simulink model "PMSMEstimate"  (R2016a)
settings: Solver=ode4  StartTime=0.0  StopTime=3  FixedStep=1e-04  RelTol=1e-3
libraries: powerlib x7, dsparch4 x7, powerlib_meascontrol x3, simulink x1
settings Model: Creator=B210b  LastModifiedBy=B210b

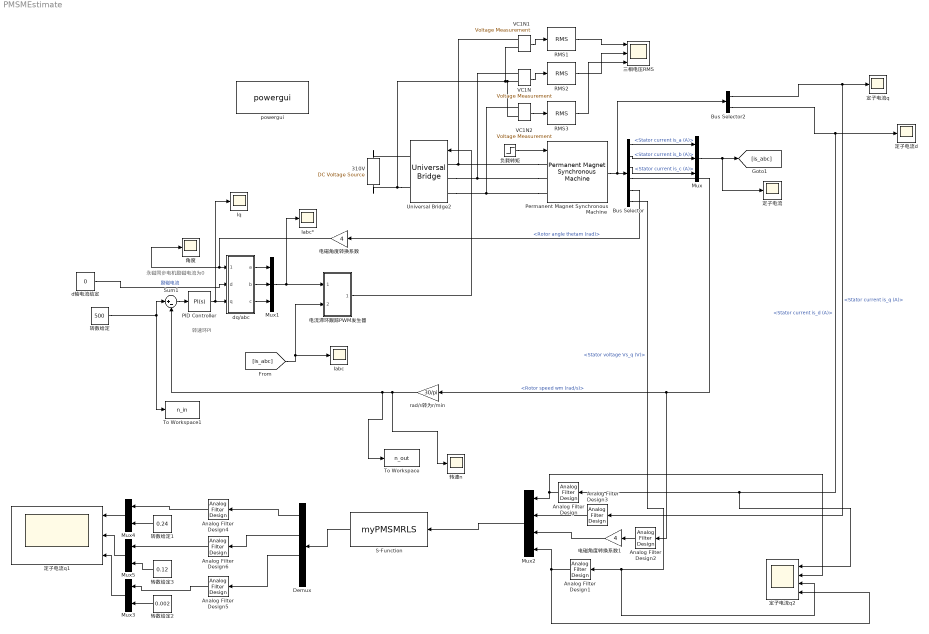
== system PMSMEstimate ==
  note: 转速环PI
  note: 永磁同步电机励磁电流为0
  310V : powerlib/Electrical Sources/DC Voltage Source  Amplitude=310  Measurements=None
  Analog Filter Design{,1..3} (4 alike) : dsparch4/Analog Filter Design  method=Butterworth  filttype=Lowpass  N=8  Wlo=50  Whi=80  Rp=2  Rs=40
  Analog Filter Design4 : dsparch4/Analog Filter Design  method=Butterworth  filttype=Lowpass  N=8  Wlo=20  Whi=80  Rp=2  Rs=40
  Analog Filter Design5 : dsparch4/Analog Filter Design  method=Butterworth  filttype=Lowpass  N=8  Wlo=20  Whi=80  Rp=2  Rs=40
  Analog Filter Design6 : dsparch4/Analog Filter Design  method=Butterworth  filttype=Lowpass  N=8  Wlo=20  Whi=80  Rp=2  Rs=40
  Bus Selector : BusSelector  OutputSignals=Stator current is_a (A),Stator current is_b (A),Stator current is_c (A),Rotor speed wm (rad/s),Rotor angle thetam (rad),Stator voltage Vs_q (V)
  Bus Selector2 : BusSelector  OutputSignals=Stator current is_q (A),Stator current is_d (A)
  Demux : Demux
  Iabc : Scope
  Iabc* : Scope
  Iq : Scope
  Mux : Mux  Inputs=3
  Mux1 : Mux  Inputs=3
  Mux2 : Mux
  Mux3 : Mux  Inputs=2
  Mux4 : Mux  Inputs=2
  Mux5 : Mux  Inputs=2
  PID Controller : simulink/Continuous/PID Controller  Controller=PI  TimeDomain=Continuous-time  SampleTime=-1  IntegratorMethod=Forward Euler  FilterMethod=Forward Euler  Form=Parallel  UseFilter=on  ControllerParametersSource=internal  P=0.05  I=8  D=0  N=100  InitialConditionSource=internal  InitialConditionForIntegrator=0  InitialConditionForFilter=0  ExternalReset=none  LimitOutput=off  UpperSaturationLimit=200  LowerSaturationLimit=-inf  LinearizeAsGain=on  AntiWindupMode=none  Kb=1  TrackingMode=off  Kt=1  PParamMin=[]  PParamMax=[]  IParamMin=[]  IParamMax=[]  DParamMin=[]  DParamMax=[]  NParamMin=[]  NParamMax=[]  KbParamMin=[]  KbParamMax=[]  KtParamMin=[]  KtParamMax=[]  POutMin=[]  POutMax=[]  IOutMin=[]  IOutMax=[]  DOutMin=[]  DOutMax=[]  NOutMin=[]  NOutMax=[]  KbOutMin=[]  KbOutMax=[]  KtOutMin=[]  KtOutMax=[]  IntegratorOutMin=[]  IntegratorOutMax=[]  FilterOutMin=[]  FilterOutMax=[]  SumOutMin=[]  SumOutMax=[]  SumI1OutMin=[]  SumI1OutMax=[]  SumI2OutMin=[]  SumI2OutMax=[]  SumI3OutMin=[]  SumI3OutMax=[]  SumDOutMin=[]  SumDOutMax=[]  SaturationOutMin=[]  SaturationOutMax=[]  IntegratorContinuousStateAttributes=''  IntegratorStateMustResolveToSignalObject=off  IntegratorRTWStateStorageClass=Auto  FilterContinuousStateAttributes=''  FilterStateMustResolveToSignalObject=off  FilterRTWStateStorageClass=Auto  DifferentiatorICPrevScaledInput=0  DifferentiatorOutMin=[]  DifferentiatorOutMax=[]
  Permanent Magnet Synchronous Machine : powerlib/Machines/Permanent Magnet Synchronous Machine  NbPhases=3  FluxDistribution=Sinusoidal  RotorType=Salient-pole  MechanicalLoad=Torque Tm  PresetModel=No  ShowDetailedParameters=on  MeasurementBus=off  Resistance=0.24  Inductance=8.5e-3  dqInductances=[0.002 0.002]  La=0.02682  MachineConstant=Flux linkage established by magnets (V.s)  Flux=0.12  VoltageCst=87.0624  TorqueCst=0.72  Flat=120  Mechanical=[0.00048 0.008 4 0]  PolePairs=2  InitialConditions=[0,0, 0,0]  InitialConditions5ph=[0 0 0 0 0 0]  TsPowergui=0  TsBlock=-1  RefAngle=Aligned with phase A axis (original Park)
  RMS1 : powerlib_meascontrol/Measurements/RMS  TrueRMS=on  Freq=100  RMSInit=0  Ts=0
  RMS2 : powerlib_meascontrol/Measurements/RMS  TrueRMS=on  Freq=100  RMSInit=0  Ts=0
  RMS3 : powerlib_meascontrol/Measurements/RMS  TrueRMS=on  Freq=100  RMSInit=0  Ts=0
  S-Function : S-Function  FunctionName=myPMSMRLS  SFunctionDeploymentMode=off  EnableBusSupport=off
  Sum1 : Sum  Inputs=|+-
  To Workspace : ToWorkspace  VariableName=n_out  SampleTime=-1
  To Workspace1 : ToWorkspace  VariableName=n_in  SampleTime=-1
  Universal Bridge2 : powerlib/Power Electronics/Universal Bridge  Arms=3  SnubberResistance=1e5  SnubberCapacitance=inf  Device=IGBT / Diodes  Ron=1e-3  Lon=0  ForwardVoltages="[  0  0  ]"  ForwardVoltage=0  GTOparameters=[ 10e-6 , 20e-6 ]  IGBTparameters=[ 1e-6 , 2e-6 ]  Measurements=None  Measurements_2=None  converterType=Rectifier
  VC1N : powerlib/Measurements/Voltage Measurement  PhasorSimulation=off  OutputType=Complex  PSBequivalent=0
  VC1N1 : powerlib/Measurements/Voltage Measurement  PhasorSimulation=off  OutputType=Complex  PSBequivalent=0
  VC1N2 : powerlib/Measurements/Voltage Measurement  PhasorSimulation=off  OutputType=Complex  PSBequivalent=0
  dq/abc : Subsystem
  d轴电流给定 : Constant  Value=0
  powergui : powerlib/powergui  SimulationMode=Continuous  SolverType=Tustin/Backward Euler (TBE)  SampleTime=0.00001  frequency=50  SPID=on  DisableSnubberDevices=off  DisableRonSwitches=off  DisableVfSwitches=off  SwTol=0  DisplayEquations=off  Interpol=off  ExternalGateDelay=off  methode=off  Ts=100  FunctionMessages=off  echomessages=off  HookPort=off  EnableUseOfTLC=off  x0status=zero  frequencyindice=0  Pbase=100e6  ErrMax=1e-4  Iterations=50  UnitsV=kV  UnitsW=MW  buscounter=0  RestoreLinks=warning  ResistiveCurrentMeasurement=off  Frange=[0:2:500]  Ylog=off  Xlog=on  ShowGrid=off  save=off  variable=ZData  structure=0  ZoomFFT=on  StartTime=0.0  cycles=1  DisplayStyle=1  fundamental=60  FreqAxis=off  MaxFrequency=1000  frequencyindicesteady=1  RmsSteady=1  display=off
  rad/s转为r/min : Gain  Gain=30/pi
  三相电压RMS : Scope  NumInputPorts=3
  定子电流 : Scope
  定子电流d : Scope
  定子电流q : Scope
  定子电流q1 : Scope  NumInputPorts=3
  定子电流q2 : Scope  NumInputPorts=4
  电流滞环跟踪PWM发生器 : Subsystem
  电磁角度转换系数 : Gain  Gain=4
  电磁角度转换系数1 : Gain  Gain=4
  角度 : Scope
  负载转矩 : Step  Time=0.02  Before=4  After=10  SampleTime=0
  转数给定 : Constant  Value=500
  转数给定1 : Constant  Value=0.24
  转数给定2 : Constant  Value=0.002
  转数给定3 : Constant  Value=0.12
  转速n : Scope
  wires:
  负载转矩/1 -> Permanent Magnet Synchronous Machine/1
  Permanent Magnet Synchronous Machine/1 -> Bus Selector2/1, Bus Selector/1
  Bus Selector/1 -> Mux/1  "<Stator current is_a (A)>"
  Bus Selector/2 -> Mux/2  "<Stator current is_b (A)>"
  Bus Selector/3 -> Mux/3  "<Stator current is_c (A)>"
  Bus Selector/4 -> Analog Filter Design2/1, rad/s转为r/min/1  "<Rotor speed wm (rad/s)>"
  Bus Selector/5 -> 电磁角度转换系数/1  "<Rotor angle thetam (rad)>"
  转数给定/1 -> Sum1/1, To Workspace1/1
  d轴电流给定/1 -> dq/abc/2(d)  "励磁电流"
  Mux/1 -> 定子电流/1, [is_abc]
  dq/abc/1(a) -> Mux1/1
  dq/abc/2(b) -> Mux1/2
  dq/abc/3(c) -> Mux1/3
  Mux1/1 -> Iabc*/1, 电流滞环跟踪PWM发生器/1(Iabc*)
  [is_abc] -> Iabc/1, 电流滞环跟踪PWM发生器/2(Iabc)
  电磁角度转换系数/1 -> 角度/1, dq/abc/1(theta)
  电流滞环跟踪PWM发生器/1(pulse) -> Universal Bridge2/1
  Sum1/1 -> PID Controller/1
  PID Controller/1 -> Iq/1, dq/abc/3(q)
  Bus Selector2/1 -> Analog Filter Design3/1, 定子电流q/1  "<Stator current is_q (A)>"
  Bus Selector2/2 -> 定子电流q2/1, Analog Filter Design/1, 定子电流d/1  "<Stator current is_d (A)>"
  rad/s转为r/min/1 -> To Workspace/1, Sum1/2, 转速n/1
  VC1N/1 -> RMS2/1
  VC1N1/1 -> RMS1/1
  RMS1/1 -> 三相电压RMS/1
  RMS2/1 -> 三相电压RMS/2
  VC1N2/1 -> RMS3/1
  RMS3/1 -> 三相电压RMS/3
  Mux2/1 -> S-Function/1
  电磁角度转换系数1/1 -> Mux2/3
  Bus Selector/6 -> 定子电流q2/3, Analog Filter Design1/1  "<Stator voltage Vs_q (V)>"
  Demux/1 -> Analog Filter Design4/1
  Demux/2 -> Analog Filter Design6/1
  Demux/3 -> Analog Filter Design5/1
  S-Function/1 -> Demux/1
  Analog Filter Design/1 -> Mux2/1, 定子电流q2/2
  Analog Filter Design3/1 -> Mux2/2
  Analog Filter Design2/1 -> 电磁角度转换系数1/1
  Analog Filter Design1/1 -> Mux2/4, 定子电流q2/4
  Mux4/1 -> 定子电流q1/1
  Mux5/1 -> 定子电流q1/2
  Mux3/1 -> 定子电流q1/3
  Analog Filter Design4/1 -> Mux4/1
  转数给定1/1 -> Mux4/2
  转数给定3/1 -> Mux5/2
  转数给定2/1 -> Mux3/2
  Analog Filter Design5/1 -> Mux3/1
  Analog Filter Design6/1 -> Mux5/1
  connections:
  Universal Bridge2/RConn2 -- 310V/LConn1 -- VC1N2/LConn2 -- VC1N/LConn2 -- VC1N1/LConn2
  Permanent Magnet Synchronous Machine/LConn1 -- Universal Bridge2/LConn1 -- VC1N1/LConn1
  Permanent Magnet Synchronous Machine/LConn3 -- Universal Bridge2/LConn3 -- VC1N2/LConn1
  Permanent Magnet Synchronous Machine/LConn2 -- Universal Bridge2/LConn2 -- VC1N/LConn1
  310V/RConn1 -- Universal Bridge2/RConn1

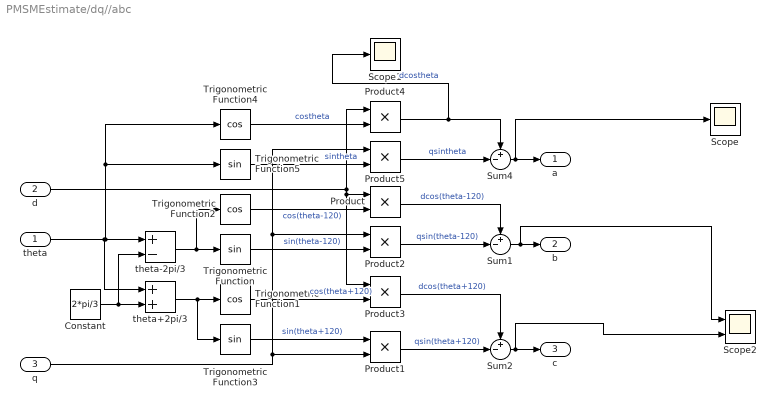
== system PMSMEstimate/dq//abc ==
  theta : Inport
  d : Inport  Port=2
  q : Inport  Port=3
  Constant : Constant  Value=2*pi/3
  Product{,1..5} (6 alike) : Product
  Scope : Scope
  Scope1 : Scope
  Scope2 : Scope  NumInputPorts=2
  Sum1 : Sum  Inputs=+-|
  Sum2 : Sum  Inputs=+-|
  Sum4 : Sum  Inputs=+-|
  Trigonometric Function : Trigonometry
  Trigonometric Function1 : Trigonometry  Operator=cos
  Trigonometric Function2 : Trigonometry  Operator=cos
  Trigonometric Function3 : Trigonometry
  Trigonometric Function4 : Trigonometry  Operator=cos
  Trigonometric Function5 : Trigonometry
  theta+2pi/3 : Sum
  theta-2pi/3 : Sum  Inputs=+-
  a : Outport
  b : Outport  Port=2
  c : Outport  Port=3
  wires:
  Trigonometric Function5/1 -> Product5/2  "sintheta"
  Product/1 -> Sum1/1  "dcos(theta-120)"
  Trigonometric Function1/1 -> Product3/2  "cos(theta+120)"
  Product3/1 -> Sum2/1  "dcos(theta+120)"
  d/1 -> Product/1, Product3/1, Product4/1
  Constant/1 -> theta+2pi/3/2, theta-2pi/3/2
  theta/1 -> Trigonometric Function4/1, Trigonometric Function5/1, theta-2pi/3/1, theta+2pi/3/1
  theta+2pi/3/1 -> Trigonometric Function3/1, Trigonometric Function1/1
  q/1 -> Product5/1, Product2/1, Product1/2
  Trigonometric Function/1 -> Product2/2  "sin(theta-120)"
  Product4/1 -> Scope1/1, Sum4/1  "dcostheta"
  Product5/1 -> Sum4/2  "qsintheta"
  theta-2pi/3/1 -> Trigonometric Function2/1, Trigonometric Function/1
  Product1/1 -> Sum2/2  "qsin(theta+120)"
  Trigonometric Function2/1 -> Product/2  "cos(theta-120)"
  Sum4/1 -> Scope/1, a/1
  Sum1/1 -> Scope2/1, b/1
  Trigonometric Function4/1 -> Product4/2  "costheta"
  Trigonometric Function3/1 -> Product1/1  "sin(theta+120)"
  Product2/1 -> Sum1/2  "qsin(theta-120)"
  Sum2/1 -> Scope2/2, c/1

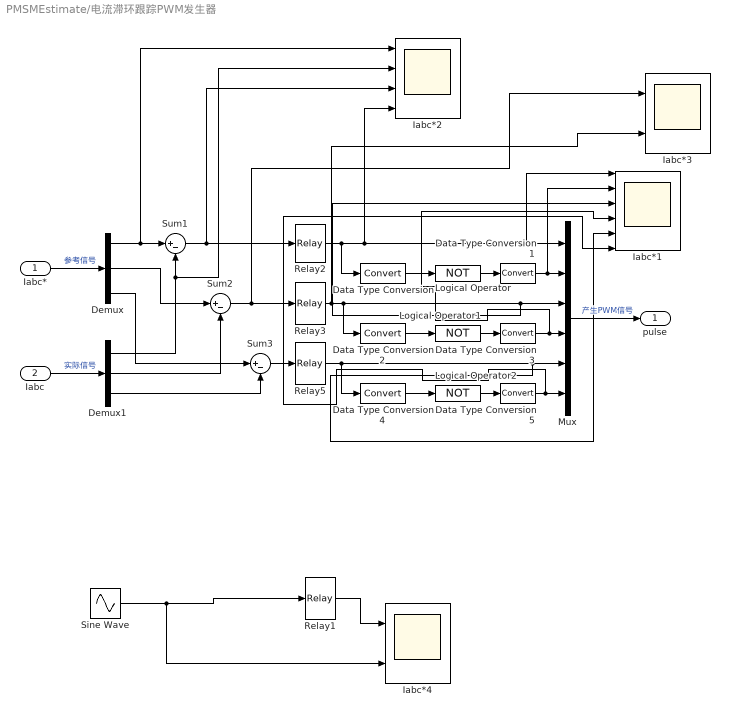
== system PMSMEstimate/电流滞环跟踪PWM发生器 ==
  Iabc* : Inport
  Iabc : Inport  Port=2
  Data Type Conversion{,1..5} (6 alike) : DataTypeConversion
  Demux : Demux  Outputs=3
  Demux1 : Demux  Outputs=3
  Iabc*1 : Scope  NumInputPorts=6
  Iabc*2 : Scope  NumInputPorts=4
  Iabc*3 : Scope  NumInputPorts=2
  Iabc*4 : Scope  NumInputPorts=2
  Logical Operator : Logic  Operator=NOT  Inputs=1  AllPortsSameDT=off
  Logical Operator1 : Logic  Operator=NOT  Inputs=1  AllPortsSameDT=off
  Logical Operator2 : Logic  Operator=NOT  Inputs=1  AllPortsSameDT=off
  Mux : Mux  Inputs=6
  Relay1 : Relay  OnSwitchValue=1  OffSwitchValue=-1  ZeroCross=off
  Relay2 : Relay  OnSwitchValue=0.1  OffSwitchValue=-0.1  ZeroCross=off
  Relay3 : Relay  OnSwitchValue=0.1  OffSwitchValue=-0.1  ZeroCross=off
  Relay5 : Relay  OnSwitchValue=0.1  OffSwitchValue=-0.1  ZeroCross=off
  Sine Wave : Sin  Amplitude=2  Frequency=2000  SampleTime=0
  Sum1 : Sum  Inputs=|+-
  Sum2 : Sum  Inputs=|+-
  Sum3 : Sum  Inputs=|+-
  pulse : Outport
  wires:
  Relay2/1 -> Data Type Conversion/1, Iabc*2/4, Iabc*1/1, Mux/1
  Data Type Conversion/1 -> Logical Operator/1
  Logical Operator/1 -> Data Type Conversion1/1
  Data Type Conversion1/1 -> Iabc*1/2, Mux/2
  Mux/1 -> pulse/1  "产生PWM信号"
  Sum1/1 -> Iabc*2/3, Relay2/1
  Demux/1 -> Iabc*2/1, Sum1/1
  Demux1/3 -> Sum3/2
  Iabc/1 -> Demux1/1  "实际信号"
  Iabc*/1 -> Demux/1  "参考信号"
  Sum2/1 -> Iabc*3/1, Relay3/1
  Logical Operator1/1 -> Data Type Conversion3/1
  Data Type Conversion3/1 -> Iabc*1/4, Mux/4
  Data Type Conversion2/1 -> Logical Operator1/1
  Logical Operator2/1 -> Data Type Conversion5/1
  Data Type Conversion5/1 -> Iabc*1/6, Mux/6
  Data Type Conversion4/1 -> Logical Operator2/1
  Relay5/1 -> Data Type Conversion4/1, Iabc*1/5, Mux/5
  Sum3/1 -> Relay5/1
  Demux/2 -> Sum2/1
  Demux1/1 -> Iabc*2/2, Sum1/2
  Demux1/2 -> Sum2/2
  Demux/3 -> Sum3/1
  Relay3/1 -> Mux/3, Iabc*1/3, Data Type Conversion2/1, Iabc*3/2
  Relay1/1 -> Iabc*4/1
  Sine Wave/1 -> Iabc*4/2, Relay1/1
